simulink model "port_checker_2013B"  (R2013b)
settings: Solver=ode45  StartTime=0.0  StopTime=8  RelTol=1e-3
libraries: dspnetwork x8, rtwinlib x1
settings Model: CovModelRefEnable=off  Creator=dave  LastModifiedBy=Anony
settings DataIOCC: SaveFormat=Dataset
settings OptimizationCC: SimCompilerOptimization=off
settings DebuggingCC: UnderspecifiedInitializationDetection=Simplified  MergeDetectMultiDrivingBlocksExec=error  SolverPrmCheckMsg=none  FrameProcessingCompatibilityMsg=error
settings HardwareCC: ProdBitPerPointer=64  ProdLargestAtomicFloat=Float  ProdIntDivRoundTo=Zero  ProdEndianess=LittleEndian  ProdHWDeviceType=Specified
settings RTWCC: RTWCompilerOptimization=off
settings GRTTargetCC: TargetLangStandard=C89/C90 (ANSI)  CodeReplacementLibrary=None  GeneratePreprocessorConditionals=Use local settings  CPPClassGenCompliant=on

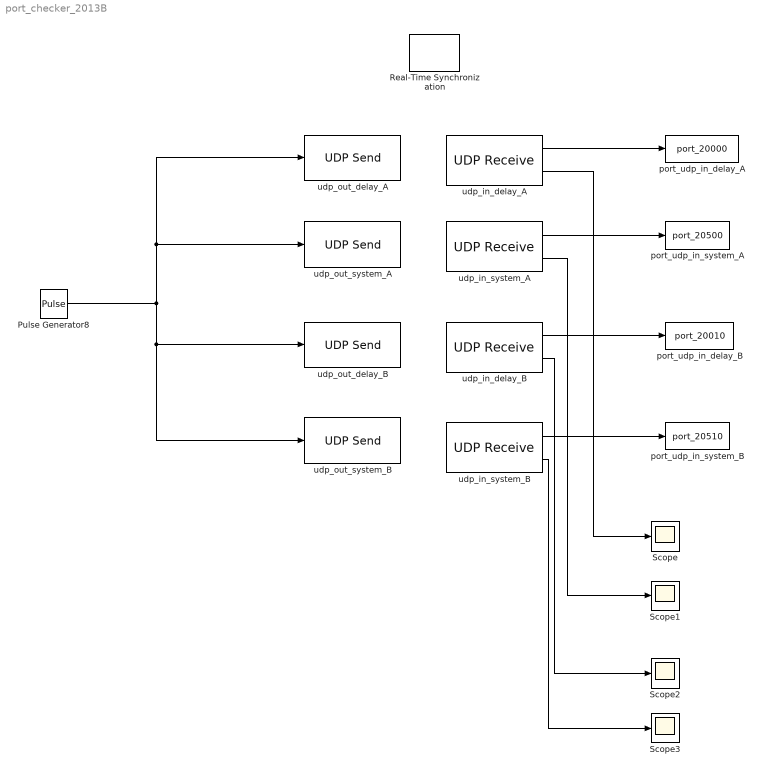
== system port_checker_2013B ==
  Pulse Generator8 : DiscretePulseGenerator  PulseType=Time based  Period=1  PulseWidth=5
  Real-Time Synchronization : rtwinlib/Real-Time Synchronization  SampleTime=0.1  MaxMissedTicks=10  ShowMissedTicks=off  YieldWhenWaiting=off
  Scope{,1..3} (4 alike) : Scope
      Scope settings: YMin=-10  YMax=10
      Scope1 settings: YMin=-10  YMax=10
      Scope2 settings: YMin=-10  YMax=10  SaveName=ScopeData2
      Scope3 settings: YMin=-10  YMax=10  SaveName=ScopeData3
  port_udp_in_delay_A : ToWorkspace  VariableName=port_20000  SampleTime=-1  SaveFormat=Timeseries
  port_udp_in_delay_B : ToWorkspace  VariableName=port_20010  SampleTime=-1  SaveFormat=Timeseries
  port_udp_in_system_A : ToWorkspace  VariableName=port_20500  SampleTime=-1  SaveFormat=Timeseries
  port_udp_in_system_B : ToWorkspace  VariableName=port_20510  SampleTime=-1  SaveFormat=Timeseries
  udp_in_delay_A : dspnetwork/UDP Receive  localURL='0.0.0.0'  localPort=20000  remoteURL='147.32.183.2'  remotePort=-1  recvBufferSize=8192  dims=255  signalDatatype=int8  isVarSize=off  showBlockingTime=off  blockingTime=0  sampletime=0.1
  udp_in_delay_B : dspnetwork/UDP Receive  localURL='0.0.0.0'  localPort=20010  remoteURL='147.32.183.2'  remotePort=-1  recvBufferSize=8192  dims=255  signalDatatype=int8  isVarSize=off  showBlockingTime=off  blockingTime=0  sampletime=0.1
  udp_in_system_A : dspnetwork/UDP Receive  localURL='0.0.0.0'  localPort=20500  remoteURL='147.32.183.2'  remotePort=-1  recvBufferSize=8192  dims=255  signalDatatype=int8  isVarSize=off  showBlockingTime=off  blockingTime=0  sampletime=0.1
  udp_in_system_B : dspnetwork/UDP Receive  localURL='0.0.0.0'  localPort=20510  remoteURL='147.32.183.2'  remotePort=-1  recvBufferSize=8192  dims=255  signalDatatype=int8  isVarSize=off  showBlockingTime=off  blockingTime=0  sampletime=0.1
  udp_out_delay_A : dspnetwork/UDP Send  remoteURL='147.32.183.2'  remotePort=21000  localURL='0.0.0.0'  localPortSource=Automatically determine  localPort=-1  sampletime=-1  separateLengthPort=0
  udp_out_delay_B : dspnetwork/UDP Send  remoteURL='147.32.183.2'  remotePort=21010  localURL='0.0.0.0'  localPortSource=Automatically determine  localPort=-1  sampletime=-1  separateLengthPort=0
  udp_out_system_A : dspnetwork/UDP Send  remoteURL='147.32.183.2'  remotePort=21500  localURL='0.0.0.0'  localPortSource=Automatically determine  localPort=-1  sampletime=-1  separateLengthPort=0
  udp_out_system_B : dspnetwork/UDP Send  remoteURL='147.32.183.2'  remotePort=21510  localURL='0.0.0.0'  localPortSource=Automatically determine  localPort=-1  sampletime=-1  separateLengthPort=0
  wires:
  Pulse Generator8/1 -> udp_out_system_B/1, udp_out_delay_B/1, udp_out_system_A/1, udp_out_delay_A/1
  udp_in_delay_A/1 -> port_udp_in_delay_A/1
  udp_in_system_B/1 -> port_udp_in_system_B/1
  udp_in_delay_B/1 -> port_udp_in_delay_B/1
  udp_in_system_A/1 -> port_udp_in_system_A/1
  udp_in_delay_A/2 -> Scope/1
  udp_in_system_A/2 -> Scope1/1
  udp_in_delay_B/2 -> Scope2/1
  udp_in_system_B/2 -> Scope3/1
